simulink model "sfcndemo_hg_gui"  (Simulink 6.0)
settings: Solver=FixedStepDiscrete  StartTime=0.0  StopTime=inf  RelTol=1e-3
settings Model: Creator=The MathWorks Inc.  LastModifiedBy=batserve  ExtModeTrigMode=oneshot  ExtModeArmWhenConnect=off  ExtModeAutoUpdateStatusClock=off
settings DataIOCC: LimitDataPoints=off
settings OptimizationCC: BlockReduction=off  BooleanDataType=off  InlineInvariantSignals=off
settings DebuggingCC: CheckExecutionContextPreStartOutputMsg=on  CheckExecutionContextRuntimeOutputMsg=on  SolverPrmCheckMsg=none
settings HardwareCC: TargetUnknown=on

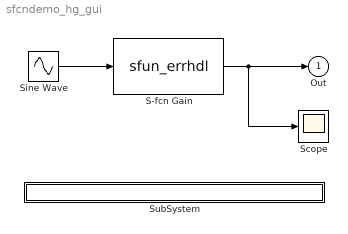
== system sfcndemo_hg_gui ==
  S-fcn Gain : S-Function  FunctionName=sfun_errhdl  Parameters=param  mask(S-function: sfun_errhdl){param=2.3}
      mask prompts: param "Input parameter:"
      mask help: An example of handling parameter checking in S-function.
      settings: DeleteFcn=sfcndemo_hg_gui_m('delete',gcbh)  NameChangeFcn=sfcndemo_hg_gui_m('namechange',gcbh)  DestroyFcn=sfcndemo_hg_gui_m('destroy',gcbh)  OpenFcn=sfcndemo_hg_gui_m('open',gcbh)  CloseFcn=sfcndemo_hg_gui_m('close',gcbh)  ParentCloseFcn=sfcndemo_hg_gui_m('parentclose',gcbh)
      mask Display: disp('HG GUI Demo');
  Scope : Scope
      settings: TickLabels=on  TimeRange=10  YMin=-10  YMax=10  DataFormat=Array
  Sine Wave : Sin  SampleTime=0
  SubSystem : Subsystem  PropExecContextAcrossSSBoundary=on
      settings: OpenFcn=edit(fullfile(matlabroot,'toolbox','simulink','simdemos','sfcndemo_hg_gui_m.m'))
      mask Display: disp('matlabroot\toolbox\simulink\simdemos\sfcndemo_hg_gui.m');
  Out : Outport  InitialOutput=0
  wires:
  Sine Wave/1 -> S-fcn Gain/1
  S-fcn Gain/1 -> Out/1, Scope/1

== system sfcndemo_hg_gui/SubSystem ==
